simulink model "TrqFactor"  (R2018b)
settings: Solver=FixedStepAuto  StartTime=0.0  StopTime=130  FixedStep=0.01  RelTol=1e-3
undefined symbols (not defined in the file or in its folder): magnitude
libraries: simulink x8
settings Model: PauseTimes=13.42  Creator=xiaoyang  LastModifiedBy=xiaoyang
settings DataIOCC: ExternalInput=[Time, Camera1__ADAS_LKAState, EPS2__EPS_SteeringTorqueValue, Camera1__ADAS_LKATorqFactReq]  LoadExternalInput=on

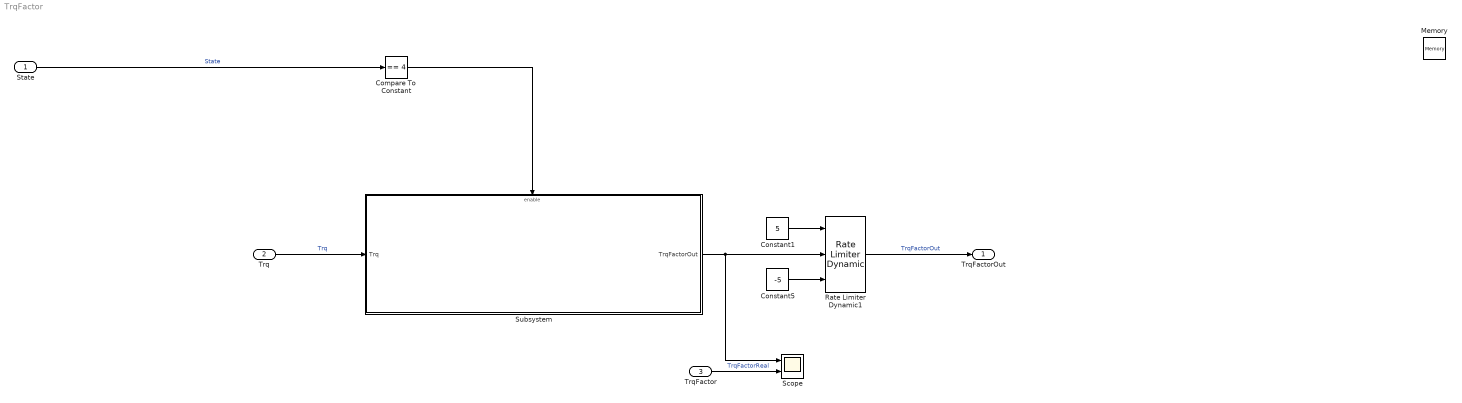
== system TrqFactor ==
  State : Inport
  Trq : Inport  Port=2
  TrqFactor : Inport  Port=3
  Compare To Constant : simulink/Logic and Bit Operations/Compare To Constant  relop===  const=4  OutDataTypeStr=boolean
  Constant1 : Constant  Value=5
  Constant5 : Constant  Value=-5
  Memory : Memory
  Rate Limiter Dynamic1 : simulink/Discontinuities/Rate Limiter Dynamic
      settings: SourceProductName=Simulink
  Scope : Scope  NumInputPorts=2
  Subsystem : Subsystem
  TrqFactorOut : Outport
  wires:
  State/1 -> Compare To Constant/1  "State"
  TrqFactor/1 -> Scope/2  "TrqFactorReal"
  Subsystem/1(TrqFactorOut) -> Rate Limiter Dynamic1/2, Scope/1
  Trq/1 -> Subsystem/1(Trq)  "Trq"
  Compare To Constant/1 -> Subsystem/Enable
  Constant5/1 -> Rate Limiter Dynamic1/3
  Constant1/1 -> Rate Limiter Dynamic1/1
  Rate Limiter Dynamic1/1 -> TrqFactorOut/1  "TrqFactorOut"

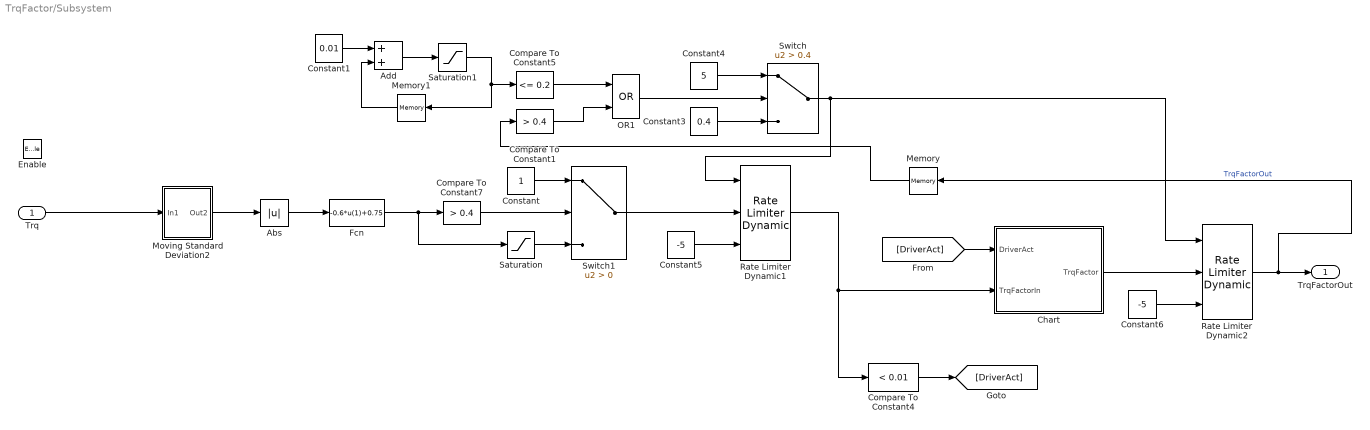
== system TrqFactor/Subsystem ==
  Trq : Inport
  Enable : EnablePort  StatesWhenEnabling=reset
  Abs : Abs
  Add : Sum
  Chart : Stateflow chart  TreatAsAtomicUnit=on
  Compare To Constant1 : simulink/Logic and Bit Operations/Compare To Constant  relop=>  const=0.4  OutDataTypeStr=boolean
  Compare To Constant4 : simulink/Logic and Bit Operations/Compare To Constant  relop=<  const=0.01  OutDataTypeStr=boolean
  Compare To Constant5 : simulink/Logic and Bit Operations/Compare To Constant  relop=<=  const=0.2  OutDataTypeStr=boolean
  Compare To Constant7 : simulink/Logic and Bit Operations/Compare To Constant  relop=>  const=0.4  OutDataTypeStr=boolean
  Constant : Constant
  Constant1 : Constant  Value=0.01
  Constant3 : Constant  Value=0.4
  Constant4 : Constant  Value=5
  Constant5 : Constant  Value=-5
  Constant6 : Constant  Value=-5
  Fcn : Fcn  Expr=-0.6*u(1)+0.75
  Memory : Memory
  Memory1 : Memory
  Moving Standard Deviation2 : Subsystem  TreatAsAtomicUnit=on
      mask Display: disp(['Moving' char(10) 'Standard' char(10) 'Deviation']);
  OR1 : Logic  Operator=OR  AllPortsSameDT=off  OutDataTypeStr=boolean
  Rate Limiter Dynamic1 : simulink/Discontinuities/Rate Limiter Dynamic
      settings: SourceProductName=Simulink
  Rate Limiter Dynamic2 : simulink/Discontinuities/Rate Limiter Dynamic
      settings: SourceProductName=Simulink
  Saturation : Saturate  UpperLimit=0.4  LowerLimit=0
  Saturation1 : Saturate  UpperLimit=0.3
  Switch : Switch  Criteria=u2 > Threshold  Threshold=0.4
  Switch1 : Switch  Criteria=u2 > Threshold
  TrqFactorOut : Outport  OutputWhenDisabled=reset  InitialOutput=0
  wires:
  Saturation/1 -> Switch1/3
  Rate Limiter Dynamic1/1 -> Compare To Constant4/1, Chart/2(TrqFactorIn)
  Fcn/1 -> Saturation/1, Compare To Constant7/1
  [DriverAct] -> Chart/1(DriverAct)
  Constant3/1 -> Switch/3
  Constant/1 -> Switch1/1
  Compare To Constant5/1 -> OR1/1
  Memory1/1 -> Add/2
  Constant4/1 -> Switch/1
  Switch1/1 -> Rate Limiter Dynamic1/2
  Compare To Constant4/1 -> [DriverAct]
  Compare To Constant7/1 -> Switch1/2
  Constant5/1 -> Rate Limiter Dynamic1/3
  Rate Limiter Dynamic2/1 -> Memory/1, TrqFactorOut/1  "TrqFactorOut"
  Constant6/1 -> Rate Limiter Dynamic2/3
  Trq/1 -> Moving Standard Deviation2/1(In1)
  Saturation1/1 -> Memory1/1, Compare To Constant5/1
  Abs/1 -> Fcn/1
  OR1/1 -> Switch/2
  Chart/1(TrqFactor) -> Rate Limiter Dynamic2/2
  Switch/1 -> Rate Limiter Dynamic2/1, Rate Limiter Dynamic1/1
  Add/1 -> Saturation1/1
  Constant1/1 -> Add/1
  Compare To Constant1/1 -> OR1/2
  Memory/1 -> Compare To Constant1/1
  Moving Standard Deviation2/1(Out2) -> Abs/1

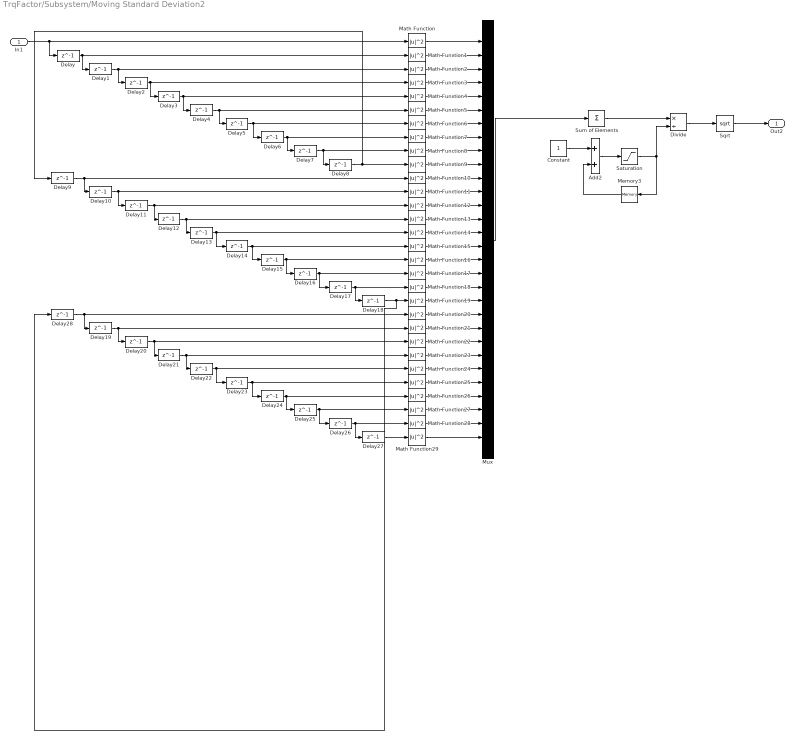
== system TrqFactor/Subsystem/Moving Standard Deviation2 ==
  In1 : Inport
  Add2 : Sum
  Constant : Constant
  Delay{,1..28} (29 alike) : Delay  DelayLength=1
  Divide : Product  Inputs=*/
  Math Function{,1..29} (30 alike) : Math  Operator=magnitude^2  SaturateOnIntegerOverflow=on
  Memory3 : Memory  InheritSampleTime=on
  Mux : Mux  Inputs=30
  Saturation : Saturate  UpperLimit=30  LowerLimit=1
      settings: AttributesFormatString="Min = %<LowerLimit>  Max = %<UpperLimit>"
  Sqrt : Sqrt  SaturateOnIntegerOverflow=on
  Sum of Elements : Sum  Inputs=+  OutDataTypeStr=Inherit: Same as first input
  Out2 : Outport
  wires:
  In1/1 -> Math Function/1, Delay/1
  Delay2/1 -> Math Function3/1, Delay3/1
  Delay1/1 -> Math Function2/1, Delay2/1
  Mux/1 -> Sum of Elements/1
  Delay/1 -> Math Function1/1, Delay1/1
  Delay3/1 -> Math Function4/1, Delay4/1
  Delay4/1 -> Math Function5/1, Delay5/1
  Delay7/1 -> Math Function8/1, Delay8/1
  Delay6/1 -> Math Function7/1, Delay7/1
  Delay5/1 -> Math Function6/1, Delay6/1
  Delay8/1 -> Delay9/1, Math Function9/1
  Delay18/1 -> Math Function19/1, Delay28/1
  Delay15/1 -> Math Function16/1, Delay16/1
  Delay16/1 -> Math Function17/1, Delay17/1
  Delay17/1 -> Math Function18/1, Delay18/1
  Delay14/1 -> Math Function15/1, Delay15/1
  Delay13/1 -> Math Function14/1, Delay14/1
  Delay10/1 -> Math Function11/1, Delay11/1
  Delay11/1 -> Math Function12/1, Delay12/1
  Delay12/1 -> Math Function13/1, Delay13/1
  Delay9/1 -> Math Function10/1, Delay10/1
  Delay28/1 -> Math Function20/1, Delay19/1
  Delay21/1 -> Math Function23/1, Delay22/1
  Delay20/1 -> Math Function22/1, Delay21/1
  Delay19/1 -> Math Function21/1, Delay20/1
  Delay22/1 -> Math Function24/1, Delay23/1
  Delay23/1 -> Math Function25/1, Delay24/1
  Delay26/1 -> Math Function28/1, Delay27/1
  Delay25/1 -> Math Function27/1, Delay26/1
  Delay24/1 -> Math Function26/1, Delay25/1
  Delay27/1 -> Math Function29/1
  Add2/1 -> Saturation/1
  Constant/1 -> Add2/1
  Memory3/1 -> Add2/2
  Sum of Elements/1 -> Divide/1
  Saturation/1 -> Divide/2, Memory3/1
  Divide/1 -> Sqrt/1
  Math Function/1 -> Mux/1
  Math Function1/1 -> Mux/2
  Math Function2/1 -> Mux/3
  Math Function3/1 -> Mux/4
  Math Function4/1 -> Mux/5
  Math Function5/1 -> Mux/6
  Math Function7/1 -> Mux/8
  Math Function6/1 -> Mux/7
  Math Function9/1 -> Mux/10
  Math Function8/1 -> Mux/9
  Math Function10/1 -> Mux/11
  Math Function11/1 -> Mux/12
  Math Function13/1 -> Mux/14
  Math Function16/1 -> Mux/17
  Math Function12/1 -> Mux/13
  Math Function14/1 -> Mux/15
  Math Function15/1 -> Mux/16
  Math Function17/1 -> Mux/18
  Math Function18/1 -> Mux/19
  Math Function23/1 -> Mux/24
  Math Function21/1 -> Mux/22
  Math Function22/1 -> Mux/23
  Math Function20/1 -> Mux/21
  Math Function28/1 -> Mux/29
  Math Function29/1 -> Mux/30
  Math Function27/1 -> Mux/28
  Math Function26/1 -> Mux/27
  Math Function24/1 -> Mux/25
  Math Function25/1 -> Mux/26
  Math Function19/1 -> Mux/20
  Sqrt/1 -> Out2/1

== stateflow chart TrqFactor/Subsystem/Chart ==
  state DriverAct
    en:
    TrqFactor = 0;
    du:
    TrqFactor = 0;
  state ADASAct
    en:
    TrqFactor = TrqFactorIn;
    du:
    TrqFactor = TrqFactorIn;
  (default) -> (junction 2)
  (junction 2) -> ADASAct [order 2]
  (junction 2) -> DriverAct [order 1] : [DriverAct == 1]
  DriverAct -> ADASAct : [DriverAct == 0 & after(1,sec)]
  ADASAct -> DriverAct : [DriverAct == 1]
  data: DriverAct input; TrqFactorIn input; TrqFactor output
